simulink model "Observer"  (R2020a)
settings: Solver=FixedStepAuto  StartTime=0.0  StopTime=10.0  FixedStep=DT  RelTol=1e-3
values from neighbouring files (symbols this model uses):
  A_aa = [-C_d/J_r C_d/J_r; C_d/(g*J_g) -C_d/(g*J_g)]    [run_Top_Model.m]
  A_ab = [-K_d/(m*J_r) s/J_r; K_d/(m*g*J_g) 0]    [run_Top_Model.m]
  A_aug = [-C_d/J_r -K_d/(m*J_r) C_d/J_r s/J_r; m 0 -m 0; C_d/(g*J_g) K_d/(m*g*J_g) -C_d/(g*J_g) 0; 0 0 0 0]    [run_Top_Model.m]
  A_ba = [m -m; 0 0]    [run_Top_Model.m]
  A_bb = [0 0; 0 0]    [run_Top_Model.m]
  A_PI = [-C_d/J_r -K_d/(m*J_r) C_d/J_r; m 0 -m; C_d/(g*J_g) K_d/(m*g*J_g) -C_d/(g*J_g)]    [run_Top_Model.m]
  B_a = [0; -s/(g*J_g)]    [run_Top_Model.m]
  B_A_PI = [s/J_r; 0; 0]    [run_Top_Model.m]
  B_aug = [0; 0; -s/(g*J_g); 0]    [run_Top_Model.m]
  B_b = [0; 0]    [run_Top_Model.m]
  B_G_PI = [0; 0; -s/(g*J_g)]    [run_Top_Model.m]
  gamma = (M_a(Omega_r_star + d_Omega_r, vx0, 0)         - M_a(Omega_r_star, vx0, 0)) / d_Omega_r    [eq_region2.m]    (also in eq_region3_cont.m = (M_a(Omega_r_star + d_Omega_r, vx0, theta_star)         - M_; run_Top_Model.m = 500)
  ini_torque = 0    [run_Top_Model.m]
  ini_wind_speed = 0    [run_Top_Model.m]
  K_i = L_kalman_PI(4)    [run_Top_Model.m]
  K_p = 50    [run_Top_Model.m]
  L_kalman_PI = L_kalman_PI(1:3)    [run_Top_Model.m]
  L_unknown = 10    [run_Top_Model.m]
  m = size(B, 2)    [eor_solve.m]    (also in regression.m = 2000; run_Top_Model.m = 1000)
  Omega_g_0 = 1    [run_Top_Model.m]
  Omega_r_0 = 1    [run_Top_Model.m]
  phi_0 = 0    [run_Top_Model.m]
  R = 63    [run_Top_Model.m]
  s = tf('s')    [baseline_design.m]    (also in eor_solve.m = size(S, 1); run_Top_Model.m = 1000000)
  tp = turbine_params_5MW()    [baseline_design.m]    (also in run_Top_Model.m)
undefined symbols (not defined in the file or in its folder): L_kal_red, L_kalman
settings Model: Creator=lpwoolcock  LastModifiedBy=lpwoolcock

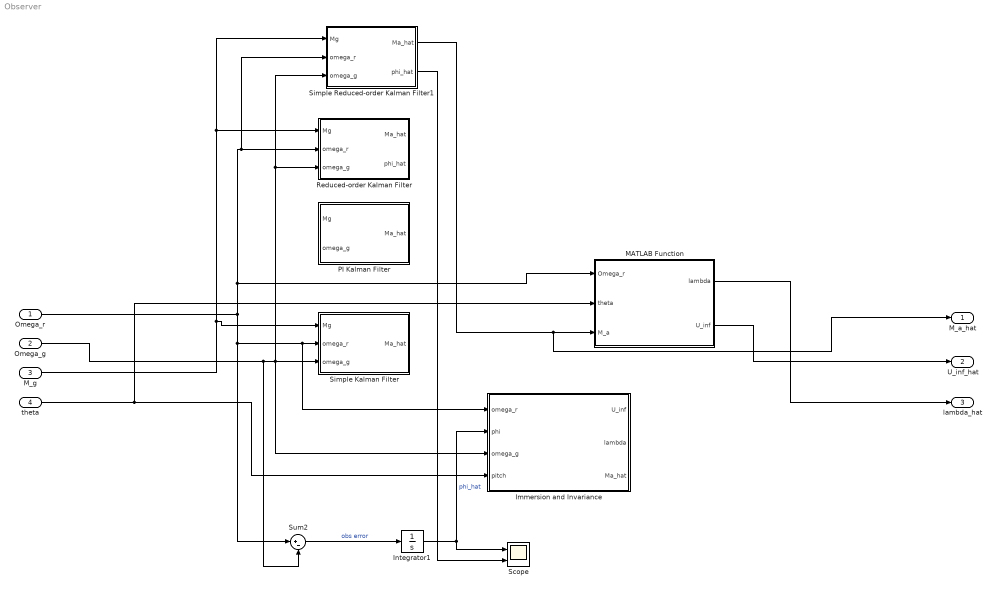
== system Observer ==
  Omega_r : Inport
  Omega_g : Inport  Port=2
  M_g : Inport  Port=3
  theta : Inport  Port=4
  Immersion and Invariance : Subsystem  TreatAsAtomicUnit=on
  Integrator1 : Integrator
  MATLAB Function : MATLAB Function  TreatAsAtomicUnit=on
  PI Kalman Filter : Subsystem  TreatAsAtomicUnit=on
  Reduced-order Kalman Filter : Subsystem  TreatAsAtomicUnit=on
  Scope : Scope  NumInputPorts=2
  Simple Kalman Filter : Subsystem  TreatAsAtomicUnit=on
  Simple Reduced-order Kalman Filter1 : Subsystem  TreatAsAtomicUnit=on
  Sum2 : Sum  Inputs=|+-
  M_a_hat : Outport
  U_inf_hat : Outport  Port=2
  lambda_hat : Outport  Port=3
  wires:
  M_g/1 -> Reduced-order Kalman Filter/1(Mg), Simple Reduced-order Kalman Filter1/1(Mg), Simple Kalman Filter/1(Mg)
  Simple Reduced-order Kalman Filter1/2(phi_hat) -> Scope/2
  Simple Reduced-order Kalman Filter1/1(Ma_hat) -> M_a_hat/1, MATLAB Function/3(M_a)
  Omega_r/1 -> Sum2/1, Immersion and Invariance/1(omega_r), Simple Kalman Filter/2(omega_r), Reduced-order Kalman Filter/2(omega_r), Simple Reduced-order Kalman Filter1/2(omega_r), MATLAB Function/1(Omega_r)
  Sum2/1 -> Integrator1/1  "obs error"
  Omega_g/1 -> Sum2/2, Reduced-order Kalman Filter/3(omega_g), Simple Reduced-order Kalman Filter1/3(omega_g), Simple Kalman Filter/3(omega_g), Immersion and Invariance/3(omega_g)
  MATLAB Function/2(U_inf) -> U_inf_hat/1
  theta/1 -> MATLAB Function/2(theta), Immersion and Invariance/4(pitch)
  MATLAB Function/1(lambda) -> lambda_hat/1
  Integrator1/1 -> Immersion and Invariance/2(phi), Scope/1  "phi_hat"

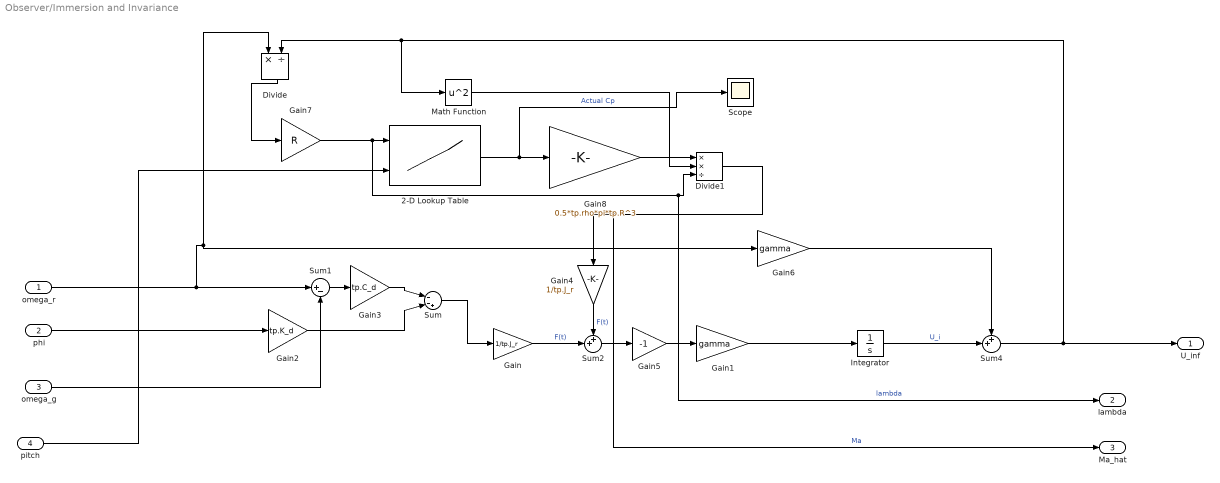
== system Observer/Immersion and Invariance ==
  omega_r : Inport
  phi : Inport  Port=2
  omega_g : Inport  Port=3
  pitch : Inport  Port=4
  2-D Lookup Table : Lookup_n-D  BreakpointsForDimension1=tp.lambda_bp  BreakpointsForDimension2=tp.theta_bp  Table=tp.C_p  InterpMethod=Cubic spline  ExtrapMethod=Cubic spline  InternalRulePriority=Speed  RndMeth=Simplest  InputSameDT=on
  Divide : Product  Inputs=*/
  Divide1 : Product  Inputs=**/
  Gain : Gain  Gain=1/tp.J_r
  Gain1 : Gain  Gain=gamma
  Gain2 : Gain  Gain=tp.K_d
  Gain3 : Gain  Gain=tp.C_d
  Gain4 : Gain  Gain=1/tp.J_r
  Gain5 : Gain  Gain=-1
  Gain6 : Gain  Gain=gamma
  Gain7 : Gain  Gain=R
  Gain8 : Gain  Gain=0.5*tp.rho*pi*tp.R^3
  Integrator : Integrator  InitialCondition=ini_wind_speed
  Math Function : Math  Operator=square  SaturateOnIntegerOverflow=on
  Scope : Scope
  Sum : Sum  Inputs=|--+
  Sum1 : Sum  Inputs=|+-
  Sum2 : Sum  Inputs=++|
  Sum4 : Sum  Inputs=++|
  U_inf : Outport
  lambda : Outport  Port=2
  Ma_hat : Outport  Port=3
  wires:
  phi/1 -> Gain2/1
  Gain2/1 -> Sum/2
  omega_g/1 -> Sum1/2
  Sum1/1 -> Gain3/1
  Gain3/1 -> Sum/1
  Sum/1 -> Gain/1
  omega_r/1 -> Sum1/1, Gain6/1, Divide/1
  Gain/1 -> Sum2/2  "F(t)"
  Gain4/1 -> Sum2/1  "F(t)"
  Sum2/1 -> Gain5/1
  Gain5/1 -> Gain1/1
  Integrator/1 -> Sum4/2  "U_i"
  Gain1/1 -> Integrator/1
  Gain6/1 -> Sum4/1
  pitch/1 -> 2-D Lookup Table/2
  Gain7/1 -> lambda/1, Divide1/3, 2-D Lookup Table/1  "lambda"
  Divide/1 -> Gain7/1
  Gain8/1 -> Divide1/1
  Divide1/1 -> Ma_hat/1, Gain4/1  "Ma"
  Math Function/1 -> Divide1/2
  2-D Lookup Table/1 -> Scope/1, Gain8/1  "Actual Cp"
  Sum4/1 -> Math Function/1, Divide/2, U_inf/1

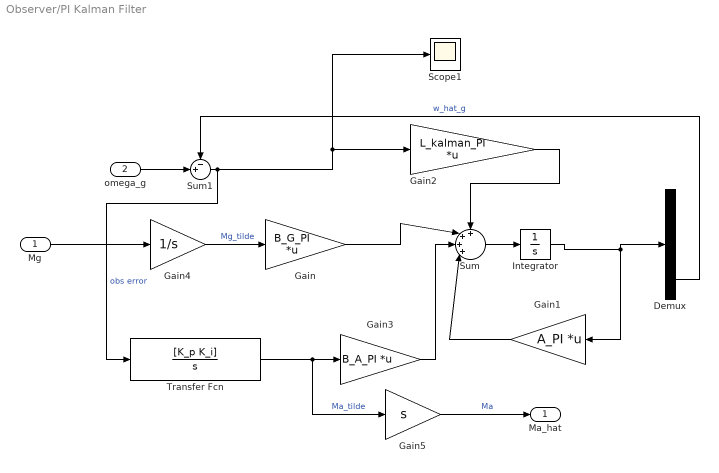
== system Observer/PI Kalman Filter ==
  Mg : Inport
  omega_g : Inport  Port=2
  Demux : Demux  Outputs=3
  Gain : Gain  Gain=B_G_PI  Multiplication=Matrix(K*u) (u vector)
  Gain1 : Gain  Gain=A_PI  Multiplication=Matrix(K*u) (u vector)
  Gain2 : Gain  Gain=L_kalman_PI  Multiplication=Matrix(K*u) (u vector)
  Gain3 : Gain  Gain=B_A_PI  Multiplication=Matrix(K*u) (u vector)
  Gain4 : Gain  Gain=1/s
  Gain5 : Gain  Gain=s
  Integrator : Integrator  InitialCondition=[Omega_r_0; phi_0; Omega_g_0]
  Scope1 : Scope
  Sum : Sum  Inputs=++++|
  Sum1 : Sum  Inputs=-+|
  Transfer Fcn : TransferFcn  Numerator=[K_p K_i]  Denominator=[1 0]
  Ma_hat : Outport
  wires:
  Mg/1 -> Gain4/1
  Sum1/1 -> Scope1/1, Gain2/1, Transfer Fcn/1  "obs error"
  Integrator/1 -> Demux/1, Gain1/1
  Gain/1 -> Sum/2
  Sum/1 -> Integrator/1
  Gain2/1 -> Sum/1
  omega_g/1 -> Sum1/2
  Gain1/1 -> Sum/4
  Demux/3 -> Sum1/1  "w_hat_g"
  Transfer Fcn/1 -> Gain5/1, Gain3/1  "Ma_tilde"
  Gain3/1 -> Sum/3
  Gain4/1 -> Gain/1  "Mg_tilde"
  Gain5/1 -> Ma_hat/1  "Ma"

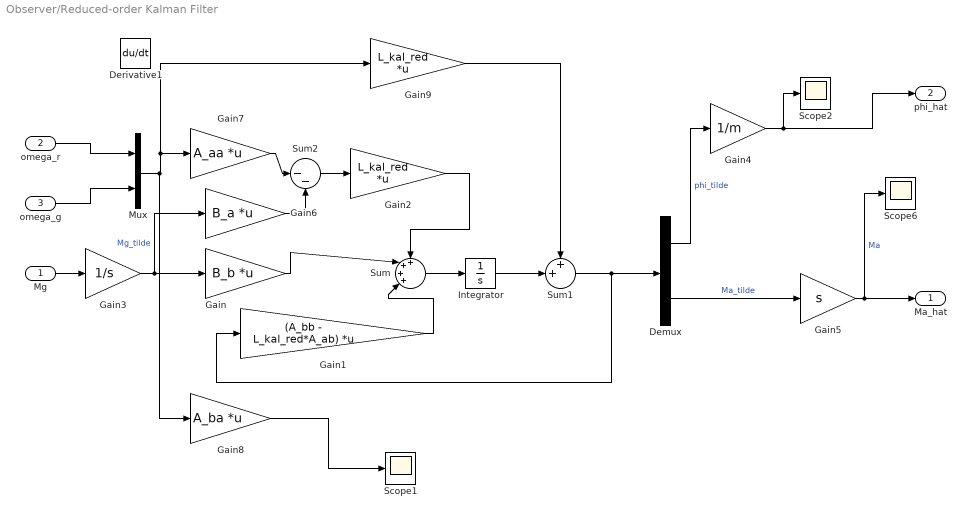
== system Observer/Reduced-order Kalman Filter ==
  Mg : Inport
  omega_r : Inport  Port=2
  omega_g : Inport  Port=3
  Demux : Demux  Outputs=2
  Derivative1 : Derivative
  Gain : Gain  Gain=B_b  Multiplication=Matrix(K*u) (u vector)
  Gain1 : Gain  Gain=(A_bb - L_kal_red*A_ab)  Multiplication=Matrix(K*u) (u vector)
  Gain2 : Gain  Gain=L_kal_red  Multiplication=Matrix(K*u) (u vector)
  Gain3 : Gain  Gain=1/s
  Gain4 : Gain  Gain=1/m
  Gain5 : Gain  Gain=s
  Gain6 : Gain  Gain=B_a  Multiplication=Matrix(K*u) (u vector)
  Gain7 : Gain  Gain=A_aa  Multiplication=Matrix(K*u) (u vector)
  Gain8 : Gain  Gain=A_ba  Multiplication=Matrix(K*u) (u vector)
  Gain9 : Gain  Gain=L_kal_red  Multiplication=Matrix(K*u) (u vector)
  Integrator : Integrator  InitialCondition=[phi_0; ini_torque]
  Mux : Mux  Inputs=2
  Scope1 : Scope
  Scope2 : Scope
  Scope6 : Scope
  Sum : Sum  Inputs=++++|
  Sum1 : Sum  Inputs=++|
  Sum2 : Sum  Inputs=|--
  Ma_hat : Outport
  phi_hat : Outport  Port=2
  wires:
  Mg/1 -> Gain3/1
  omega_r/1 -> Mux/1
  omega_g/1 -> Mux/2
  Demux/2 -> Gain5/1  "Ma_tilde"
  Gain/1 -> Sum/2
  Gain1/1 -> Sum/4
  Sum/1 -> Integrator/1
  Gain3/1 -> Gain6/1, Gain/1  "Mg_tilde"
  Gain5/1 -> Scope6/1, Ma_hat/1  "Ma"
  Gain2/1 -> Sum/1
  Gain4/1 -> phi_hat/1, Scope2/1
  Demux/1 -> Gain4/1  "phi_tilde"
  Sum1/1 -> Gain1/1, Demux/1
  Integrator/1 -> Sum1/2
  Sum2/1 -> Gain2/1
  Mux/1 -> Gain8/1, Gain9/1, Gain7/1
  Gain8/1 -> Scope1/1
  Gain6/1 -> Sum2/2
  Gain7/1 -> Sum2/1
  Gain9/1 -> Sum1/1

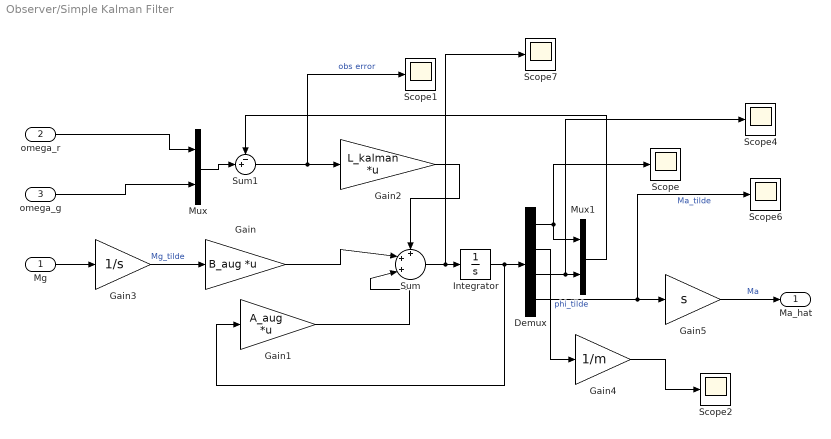
== system Observer/Simple Kalman Filter ==
  Mg : Inport
  omega_r : Inport  Port=2
  omega_g : Inport  Port=3
  Demux : Demux
  Gain : Gain  Gain=B_aug  Multiplication=Matrix(K*u) (u vector)
  Gain1 : Gain  Gain=A_aug  Multiplication=Matrix(K*u) (u vector)
  Gain2 : Gain  Gain=L_kalman  Multiplication=Matrix(K*u) (u vector)
  Gain3 : Gain  Gain=1/s
  Gain4 : Gain  Gain=1/m
  Gain5 : Gain  Gain=s
  Integrator : Integrator  InitialCondition=[Omega_r_0; Omega_g_0; phi_0; ini_torque]
  Mux : Mux  Inputs=2
  Mux1 : Mux  Inputs=2
  Scope{,1..2,4,6..7} (6 alike) : Scope
  Sum : Sum  Inputs=+++|
  Sum1 : Sum  Inputs=-+|
  Ma_hat : Outport
  wires:
  Mg/1 -> Gain3/1
  omega_r/1 -> Mux/1
  omega_g/1 -> Mux/2
  Mux/1 -> Sum1/2
  Sum1/1 -> Scope1/1, Gain2/1  "obs error"
  Integrator/1 -> Gain1/1, Demux/1
  Demux/4 -> Scope6/1, Gain5/1  "Ma_tilde"
  Gain/1 -> Sum/2
  Gain1/1 -> Sum/3
  Sum/1 -> Scope7/1, Integrator/1
  Demux/3 -> Scope4/1, Mux1/2
  Demux/1 -> Scope/1, Mux1/1
  Mux1/1 -> Sum1/1
  Demux/2 -> Gain4/1  "phi_tilde"
  Gain3/1 -> Gain/1  "Mg_tilde"
  Gain5/1 -> Ma_hat/1  "Ma"
  Gain2/1 -> Sum/1
  Gain4/1 -> Scope2/1

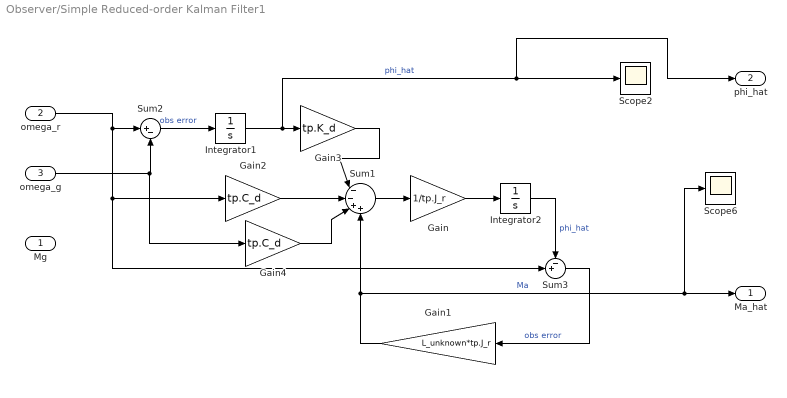
== system Observer/Simple Reduced-order Kalman Filter1 ==
  Mg : Inport
  omega_r : Inport  Port=2
  omega_g : Inport  Port=3
  Gain : Gain  Gain=1/tp.J_r
  Gain1 : Gain  Gain=L_unknown*tp.J_r
  Gain2 : Gain  Gain=tp.C_d
  Gain3 : Gain  Gain=tp.K_d
  Gain4 : Gain  Gain=tp.C_d
  Integrator1 : Integrator
  Integrator2 : Integrator
  Scope2 : Scope
  Scope6 : Scope
  Sum1 : Sum  Inputs=|--++
  Sum2 : Sum  Inputs=|+-
  Sum3 : Sum  Inputs=-+|
  Ma_hat : Outport
  phi_hat : Outport  Port=2
  wires:
  omega_r/1 -> Gain2/1, Sum3/2, Sum2/1
  omega_g/1 -> Gain4/1, Sum2/2
  Gain1/1 -> Scope6/1, Ma_hat/1, Sum1/4  "Ma"
  Sum2/1 -> Integrator1/1  "obs error"
  Sum1/1 -> Gain/1
  Gain/1 -> Integrator2/1
  Integrator2/1 -> Sum3/1  "phi_hat"
  Sum3/1 -> Gain1/1  "obs error"
  Gain2/1 -> Sum1/2
  Integrator1/1 -> phi_hat/1, Scope2/1, Gain3/1  "phi_hat"
  Gain3/1 -> Sum1/1
  Gain4/1 -> Sum1/3

== matlab function Observer/MATLAB Function ==
  data: Omega_r input; theta input; lambda output; M_a input; U_inf output; tp parameter Bus: slBus1
% Computes the windspeed using a secant method with given torque
% estimation, rotor speed, and blade pitch angle
function [lambda, U_inf] = torque_to_windspeed(Omega_r, theta, M_a, tp)

C = 2*M_a/(tp.rho*pi*tp.R^5*(Omega_r)^2);
% Root finding using secant method

% initial guesses for lambda, assume we lie close to optimal
x_n_1 = 0.9*tp.lambda_star; %x[n]
x_n = 1.1*tp.lambda_star; %x[n-1]

eps = 0.001; %minimal lambda movement
max_iter = 1000;
iterations = 0;
delta_x = x_n - x_n_1; %initialise initial delta;

while (abs(delta_x) > eps && iterations < max_iter)
    temp = x_n;
    Cp_val = interp2(tp.theta_grid, tp.lambda_grid, tp.C_p,...
         [theta, theta], [x_n, x_n_1]);
    %function values at previous time steps
    f_x_n = Cp_val(1)/(x_n)^3 - C;
    f_x_n_1 = Cp_val(2)/(x_n_1)^3 - C;
    
    %update new guess for lambda
    x_n = (x_n_1*f_x_n - x_n*f_x_n_1)/(f_x_n - f_x_n_1);
    x_n_1 = temp;
    delta_x = x_n - x_n_1;
    iterations = iterations + 1;
end

U_inf = tp.R*Omega_r/x_n; 
lambda = x_n;
end
